simulink model "W2ques1_stateflow"  (R2020b)
settings: Solver=VariableStepAuto  StartTime=0.0  StopTime=10.0  RelTol=1e-3
settings Model: Creator=sneha  LastModifiedBy=sneha

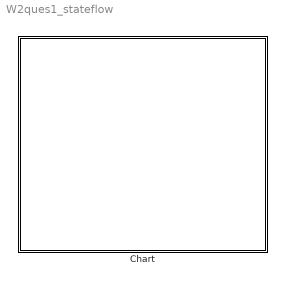
== system W2ques1_stateflow ==
  Chart : Stateflow chart  TreatAsAtomicUnit=on

== stateflow chart W2ques1_stateflow/Chart ==
  state DigitOne
    state StateZero
      entry:
      Data_d1=0;
    state StateOne
      entry:
      Data_d1=1;
    state StateFour
      entry:
      Data_d1=4;
    state StateThree
      entry:
      Data_d1=3;
    state StateTwo
      entry:
      Data_d1=2;
    (default) -> DigitOne.StateZero
    DigitOne.StateFour -> DigitOne.StateZero : after(1,sec){send(ChangeDigitTwo,DigitTwo)}
    DigitOne.StateZero -> DigitOne.StateOne : after(1,sec)
    DigitOne.StateThree -> DigitOne.StateFour : after(1,sec)
    DigitOne.StateOne -> DigitOne.StateTwo : after(1,sec)
    DigitOne.StateTwo -> DigitOne.StateThree : after(1,sec)
  state DigitTwo
    state StateZero
      entry:
      Data_d2=0;
    state StateOne
      entry:
      Data_d2=1;
    state StateFour
      entry:
      Data_d2=4;
    state StateThree
      entry:
      Data_d2=3;
    state StateTwo
      entry:
      Data_d2=2;
    (default) -> DigitTwo.StateZero
    DigitTwo.StateFour -> DigitTwo.StateZero : ChangeDigitTwo{send(ChangeDigitThree,DigitThree)}
    DigitTwo.StateZero -> DigitTwo.StateOne : ChangeDigitTwo
    DigitTwo.StateThree -> DigitTwo.StateFour : ChangeDigitTwo
    DigitTwo.StateOne -> DigitTwo.StateTwo : ChangeDigitTwo
    DigitTwo.StateTwo -> DigitTwo.StateThree : ChangeDigitTwo
  state DigitThree
    state StateZero
      entry:
      Data_d2=0;
    state StateOne
      entry:
      Data_d2=1;
    state StateFour
      entry:
      Data_d2=4;
    state StateThree
      entry:
      Data_d2=3;
    state StateTwo
      entry:
      Data_d2=2;
    (default) -> DigitThree.StateZero
    DigitThree.StateFour -> DigitThree.StateZero : ChangeDigitThree
    DigitThree.StateZero -> DigitThree.StateOne : ChangeDigitThree
    DigitThree.StateThree -> DigitThree.StateFour : ChangeDigitThree
    DigitThree.StateOne -> DigitThree.StateTwo : ChangeDigitThree
    DigitThree.StateTwo -> DigitThree.StateThree : ChangeDigitThree
